simulink model "exampleElectricHeater"  (Simulink 7.6)
settings: Solver=ode45  StartTime=0.0  StopTime=3600  MaxStep=60  RelTol=1e-3
libraries: carnot x3
settings Model: Creator=drhf  LastModifiedBy=drhf
settings CodeAppCC: CustomSymbolStrType=$N$R$M_T

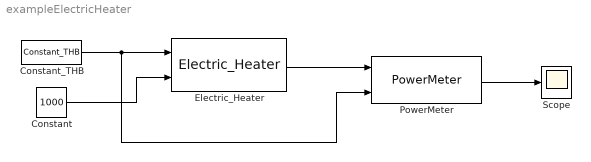
== system exampleElectricHeater ==
  Constant : Constant  Value=1000
  Constant_THB : carnot/Source/Simple/Constant_THB  SystemSampleTime=-1  t=40  mdot=500/3600  p=1e5  mID=No Pressure Drop  fluid=Water  mix=0  dia=0.02  hgt=0
  Electric_Heater : carnot/Source/Boiler/Electric_Heater  SystemSampleTime=-1
  PowerMeter : carnot/Control/PowerMeter  SystemSampleTime=-1
  Scope : Scope
  wires:
  Constant_THB/1 -> PowerMeter/2, Electric_Heater/1
  Constant/1 -> Electric_Heater/2
  Electric_Heater/1 -> PowerMeter/1
  PowerMeter/1 -> Scope/1
